simulink model "Dynamic_art25"  (R2018b)
settings: Solver=VariableStepAuto  StartTime=0.0  StopTime=10.0  RelTol=1e-3
libraries: simulink x1
settings Model: Creator=giga4  LastModifiedBy=Utente

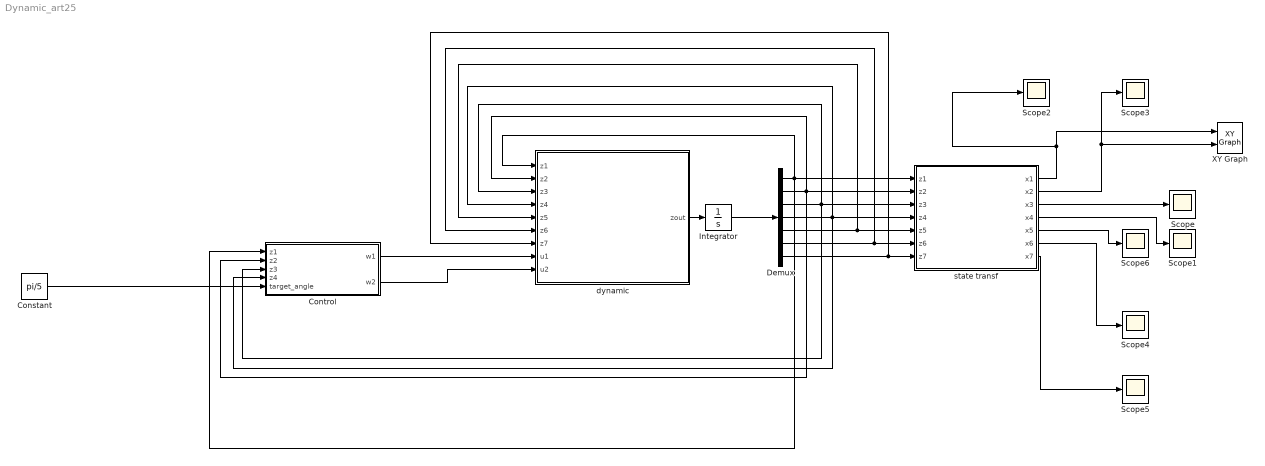
== system Dynamic_art25 ==
  Constant : Constant  Value=pi/5
  Control : MATLAB Function  TreatAsAtomicUnit=on
  Demux : Demux  Outputs=7
  Integrator : Integrator  InitialCondition=[pi;0;-pi/180;0;0;0;10]
  Scope{,1..6} (7 alike) : Scope
  XY Graph : simulink/Sinks/XY Graph  xmin=-10  xmax=10  ymin=-10  ymax=10  st=-1
  dynamic : MATLAB Function  TreatAsAtomicUnit=on
  "state transf " : MATLAB Function  TreatAsAtomicUnit=on
  wires:
  dynamic/1(zout) -> Integrator/1
  Integrator/1 -> Demux/1
  Demux/1 -> dynamic/1(z1), "state transf "/1(z1), Control/1(z1)
  Demux/2 -> "state transf "/2(z2), dynamic/2(z2), Control/2(z2)
  Demux/3 -> "state transf "/3(z3), dynamic/3(z3), Control/3(z3)
  Demux/4 -> "state transf "/4(z4), dynamic/4(z4), Control/4(z4)
  Demux/5 -> "state transf "/5(z5), dynamic/5(z5)
  Demux/6 -> "state transf "/6(z6), dynamic/6(z6)
  Demux/7 -> "state transf "/7(z7), dynamic/7(z7)
  Control/1(w1) -> dynamic/8(u1)
  Control/2(w2) -> dynamic/9(u2)
  "state transf "/3(x3) -> Scope/1
  "state transf "/4(x4) -> Scope1/1
  "state transf "/1(x1) -> Scope2/1, XY Graph/1
  "state transf "/2(x2) -> Scope3/1, XY Graph/2
  "state transf "/6(x6) -> Scope4/1
  "state transf "/7(x7) -> Scope5/1
  "state transf "/5(x5) -> Scope6/1
  Constant/1 -> Control/5(target_angle)

== matlab function Dynamic_art25/Control ==
  data: w1 output; z1 input; z2 input; z3 input; z4 input; w2 output; target_angle input
function [w1,w2] = control(z1,z2,z3,z4,target_angle)
        
    kqv = 5;
    kq = 100;
    kav = 10;
    ka = 1000;

    w1 =  -kqv*z2 - kq*(z1-target_angle) %-kqv*z2;
    w2 =  -kav*z4 - ka*(z3); %-kav*z4


end

== matlab function Dynamic_art25/dynamic ==
  data: zout output; z1 input; z2 input; z3 input; z4 input; z5 input; z6 input; z7 input; u1 input; u2 input
function zout = dynamic(z1,z2,z3,z4,z5,z6,z7,u1,u2)

%     z1 = z(1);
%     z2 = z(2);
%     z3 = z(3);
%     z4 = z(4);
%     z5 = z(5);
%     z6 = z(6);
%     z7 = z(7);

    fz = [z2; 
        0;
        z4;
        0;
        (cos(z1)*(z7 - 1.0*z4*(0.547*cos(z3) + 1.0)))/(2.19*cos(z3) + 3.11);
        (sin(z1)*(z7 - 1.0*z4*(0.547*cos(z3) + 1.0)))/(2.19*cos(z3) + 3.11);
        (2.19*cos(z3) + 3.11)*(z2^2*(1.99*sin(3.0*z3) - 6.77*sin(z3)) + (23.5*sin(2.0*z3))/(4.79*cos(z3)^2 - 12.5) - (1.0*(0.547*cos(z3) + 1.0)*((3.28*sin(2.0*z3)*z2^2)/(4.79*cos(z3)^2 - 12.5) + (173.0*sin(z3))/(4.79*cos(z3)^2 - 12.5) - (2.39*z4^2*sin(2.0*z3))/(4.79*cos(z3)^2 - 12.5)))/(2.19*cos(z3) + 3.11) - (2.19*z4^2*sin(2.0*z3))/(4.79*cos(z3)^2 - 12.5)) - 1.0*z4*(2.19*sin(z3)*(z7 - 1.0*z4*(0.547*cos(z3) + 1.0)) + 0.547*z4*sin(z3));
     ];
 
    g1z = [0;1;0;0;0;0;0];
    g2z = [0;0;0;1;0;0;0];
    input = g1z*u1 + g2z*u2;
    zout = fz + input;

end

== matlab function Dynamic_art25/state transf  ==
  data: x1 output; z1 input; z2 input; z3 input; z4 input; z5 input; z6 input; z7 input; x2 output; x3 output; x4 output; x5 output; x6 output; x7 output
function [x1,x2,x3,x4,x5,x6,x7]  = control(z1,z2,z3,z4,z5,z6,z7)
        
        x1 = z5;
        x2 = z6;
        x3 = z1;
        x4 = z3;
        x5 = z4;
        x7 = z2;
        x6 = (z7+x5*(-(35*cos(z3))/64 - 1603/1600))/(35*cos(z3))/16 + 249/80;
 

end
